simulink model "North_Country_Grid"  (R2025a)
settings: Solver=VariableStepAuto  StartTime=0.0  StopTime=10  RelTol=1e-3
PreLoadFcn:
  | Ts=50e-6;
InitFcn:
  | xInitial = WindFarmType4AverageModelInit;
  | Ts=50e-6;
undefined symbols (not defined in the file): D1, D11, Delta, DiscIntNeverNeededParam, find_system, Fnom_I, Fnom_R, Idc_nom, lagging, level, pulse, test_alpha, Vdc_nom, VLL_nom_I, VLL_nom_R
libraries: spsSecondOrderFilterLib x47, powerlib_extras x38, simulink x34, spsThreePhaseVIMeasurementLib x30, spsFirstOrderFilterLib x29, simulink_extras x26, spsabctodq0Lib x25, spsThreePhaseTransformerTwoWindingsLib x19, spsThreePhaseBreakerLib x18, spsThreePhasePISectionLineLib x17, spsControlledVoltageSourceLib x15, spsOnDelayLib x12
(part 3 of 18)

== system North_Country_Grid/Noble Ellenburg (Type 4, 81 MW) ==
  1 km collector line : spsThreePhasePISectionLineLib/Three-Phase PI Section Line  LConnTagsString=a|b|c  RConnTagsString=A|B|C  Length=1  Frequency=60  Resistances=[ 0.01273 0.3864]  Inductances="[ 0.9337e-3  4.1264e-3]"  Capacitances=[12.74e-9 7.751e-9]
  34.5 kV/ 690V 400 MVA : spsThreePhaseTransformerTwoWindingsLib/Three-Phase Transformer (Two Windings)  Winding1Connection=Delta (D11)  Winding2Connection=Yg  CoreType=Three single-phase transformers  SetSaturation=off  Hysteresis=off  DataFile='hysteresis'  SetInitialFlux=off  Measurements=None  UNITS=pu  NominalPower="[400e6  60]"  Winding1=[34.5e3 , 0.0125 , 0.025]  Winding2=[690, 0.0125, 0.025]  Rm=500  Lm=inf  L0=0.5  Saturation=[ 0,0 ; 0.0024,1.2 ; 1.0,1.52 ]  InitialFluxes=[ 0.8 , -0.8 , 0.7 ]  BreakLoop=off  DiscreteSolver=Trapezoidal iterative  DataType=off  TransfoNumber=0
  345kV/34.5 kV 400 MVA : spsThreePhaseTransformerTwoWindingsLib/Three-Phase Transformer (Two Windings)  Winding1Connection=Delta (D11)  Winding2Connection=Yg  CoreType=Three single-phase transformers  SetSaturation=off  Hysteresis=off  DataFile='basic_model'  SetInitialFlux=off  Measurements=None  UNITS=pu  NominalPower=[400e6 60 ]  Winding1="[ 345e3  0.0125   0.025 ]"  Winding2="[34.5e3  0.0125  0.025]"  Rm=500  Lm=inf  L0=0.5  Saturation="[ 0,0  ;  0.005,1.2  ;  1.0,1.4 ]"  InitialFluxes=[ 0.8 , -0.8 , 0.7 ]  BreakLoop=off  DiscreteSolver=Trapezoidal iterative  DataType=off  TransfoNumber=0
  B6 (690 V) : spsThreePhaseVIMeasurementLib/Three-Phase V-I Measurement  VoltageMeasurement=phase-to-ground  SetLabelV=on  LabelV=Vabc_B6  Vpu=on  VpuLL=off  CurrentMeasurement=yes  SetLabelI=on  LabelI=Iabc_B6  Ipu=on  Pbase=5*2e6/0.9  Vbase=690  OutputType=Complex  PhasorSimulation=off  PSBequivalent=0
  Bus Selector : BusSelector  OutputSignals=Vdc_V,wr_pu,PQ_pu.P_pu,PQ_pu.Q_pu
  Constant : Constant  Value=15
  Constant1 : Constant  Value=0
  Demux : Demux  Outputs=2
  MW : Gain  Gain=54*1.5  SaturateOnIntegerOverflow=on  OutDataTypeStr=Inherit: Same as input  ParamDataTypeStr=Inherit: Same as input
  Mux : Mux  Inputs=2
  Wind Farm : Subsystem  LoadFcn=%find_system(gcs,'FollowLinks', 'on', 'LookUnderMasks', 'all');  mask(Wind Turbine: Model 7){Nb_wt=54, ShowParameters=Control parameters for 1 wind turbine, nom=[1.5e6 690 60], Reactances=[ 1.305, 0.296, 0.252, 0.474,  0.243,  0.18 ], Time_constants=[  4.49  0.0681  0.0513  ], Resistance=0.006, mec=[0.62 0.01 1], init=[ 0  0  0  0  0  0  0  0  1 ], Vnom=690, Imax_grid_conv=1.1, RL_grid=[ 0.15 0.15/50], C_var_filter1=150e3, Vdc_nom=1100, C_DClink1=90000e-6, L_R_Boost=[0.0012     5e-3], Pmec1=2e6, wind_speed_CpMax=11, wind0=11, DisplayTurbChar=off, H_WT=4.32, Ksh=0.3, D_mutual=1.5, w_wt0=1, torque0=1, Kdc=[1.1   27.5], Ki_var_reg=0.05, Ki_volt_reg=2, Kgrid_side_cur_reg=[1  50], Kspeed=[5 1], Kboost_cur_reg=[0.025 100], Kp_pitch=15, Kcompensation=[1.5  6], Kfield=[10  20], pitch_max=27, pitch_rate=10, Ts=Ts}
      mask prompts: Nb_wt "Number of wind turbines:"; ShowParameters "Display:"; nom "Nom. power, L-L volt. and freq.: [Pn (VA), Vn (Vrms), fn (Hz)]"; Reactances "Reactances [Xd Xd' Xd'' Xq Xq'' Xl] (p.u.):"; Time_constants "Time constants [Tdo' Tdo'' Tq''] (s):"; Resistance "Resistance Rs (p.u.):"; mec "Inertia constant, friction factor, and pairs of poles: [ H(s)  F(p.u.)  p ]"; init "Initial conditions: [dw(%) th(deg) ia,ib,ic(pu) pha,phb,phc(deg) Vf(pu)]:"; Vnom "Grid-side converter nominal AC voltage (V):"; Imax_grid_conv "Grid-side converter maximum AC current (pu based on generator power and converter nominal AC voltage):"; RL_grid "Grid-side coupling inductor [ L(pu) R(pu),pu based on generator power and converter nominal AC voltage] :"; C_var_filter1 "Line filter capacitor (Q=50) (var):"; Vdc_nom "Nominal DC bus voltage (V)"; C_DClink1 "DC bus capacitor (F):"; L_R_Boost "Boost converter inductance [L(H) R(ohm)]:"; Pmec1 "Nominal mechanical output power (W):"; wind_speed_CpMax "Wind speed at nominal speed and at Cp max (must be between 6 m/s and 30 m/s) (m/s):"; wind0 "Initial wind speed (m/s):"; DisplayTurbChar "Display wind turbine power characteristics:"; H_WT "Wind turbine inertia constant H (s):"; Ksh "Shaft spring constant refer to high-speed shaft (pu of nominal mechanical torque/rad):"; D_mutual "Shaft mutual damping (pu of nominal mechanical torque/pu dw):"; w_wt0 "Turbine initial speed (pu of nominal speed):"; torque0 "Initial output torque (pu of nominal mechanical torque):"; Kdc "DC bus voltage regulator gains [Kp Ki]:"; Ki_var_reg "Grid-side converter var regulator gain [ Ki]:"; Ki_volt_reg "Grid-side converter voltage regulator gain [ Ki]:"; Kgrid_side_cur_reg "Grid-side converter current regulator gains [Kp Ki]:"; Kspeed "Speed regulator gains [Kp Ki]:"; Kboost_cur_reg "Boost inductor current regulator gains [Kp Ki]:"; Kp_pitch "Pitch controller gain [Kp]:"; Kcompensation "Pitch compensation gains [Kp Ki]:"; Kfield "Field excitation gains [Kp Ki]:"; pitch_max "Maximum pitch angle (deg):"; pitch_rate "Maximum rate of change of pitch angle (deg/s)"; Ts "Sample time (s):"
      mask help: This block implements a model of a variable speed pitch controlled wind turbine using a synchronous generator.
      mask init: same as North_Country_Grid/Marble River (Type 4, 215.25 MW)/Wind Farm
      mask TypeOptions ShowParameters: Generator data for 1 wind turbine | Converters data for 1 wind turbine | Turbine data for 1 wind turbine | Drive train data for 1 wind turbine | Control parameters for 1 wind turbine
      mask Callback ShowParameters:
      | BlockName=getfullname(gcb);
      | %
      | Param_Show=get_param(BlockName,'ShowParameters');
      | Param_DisplayTurbChar=get_param(BlockName,'DisplayTurbChar');
      | 
      | p_mask{3}='off';p_mask{4}='off';p_mask{5}='off';
      | p_mask{6}='off';p_mask{7}='off';p_mask{8}='off';p_mask{9}='off';
      | p_mask{10}='off';p_mask{11}='off';p_mask{12}='off';p_mask{13}='off';
      | p_mask{14}='off';p_mask{15}='off';p_mask{16}='off';p_mask{17}='off';
      | p_mask{18}='off';p_mask{19}='off';p_mask{20}='off';p_mask{21}='off';
      | p_mask{22}='off';p_mask{23}='off';p_mask{24}='off';p_mask{25}='off';
      | p_mask{26}='off';p_mask{27}='off';p_mask{28}='off';p_mask{29}='off';
      | p_mask{30}='off';p_mask{31}='off';p_mask{32}='off';p_mask{33}='off';
      | p_mask{34}='off';p_mask{35}='off';
      | 
      | switch Param_Show
      | 	case 'Generator data for 1 wind turbine'
      | 		p_mask{3}='on';p_mask{4}='on';p_mask{5}='on';
      |         p_mask{6}='on';p_mask{7}='on';p_mask{8}='on';
      |     case 'Converters data for 1 wind turbine'
      | 		p_mask{9}='on';p_mask{10}='on';p_mask{11}='on';
      |         p_mask{12}='on';p_mask{13}='on';p_mask{14}='on';p_mask{15}='on';
      | 	case 'Turbine data for 1 wind turbine'
      | 		p_mask{16}='on';p_mask{17}='on';p_mask{18}='on';p_mask{19}='on';
      |     case 'Drive train data for 1 wind turbine'
      |         p_mask{20}='on';p_mask{21}='on';p_mask{22}='on';p_mask{23}='on';
      |         p_mask{24}='on';
      |     case 'Control parameters for 1 wind turbine'
      |         p_mask{25}='on';p_mask{26}='on';p_mask{27}='on';
      |         p_mask{28}='on';p_mask{29}='on';p_mask{30}='on';p_mask{31}='on';
      |         p_mask{32}='on';p_mask{33}='on';p_mask{34}='on';p_mask{35}='on';
      | end
      | 
      | ParVisible={'on','on',p_mask{3},p_mask{4},p_mask{5},p_mask{6},...
      |     p_mask{7},p_mask{8},p_mask{9},p_mask{10},p_mask{11},p_mask{12},...
      |     p_mask{13},p_mask{14},p_mask{15},p_mask{16},p_mask{17},p_mask{18},...
      |     p_mask{19},p_mask{20},p_mask{21},p_mask{22},p_mask{23},p_mask{24},...
      |     p_mask{25},p_mask{26},p_mask{27},p_mask{28},p_mask{29},p_mask{30},...
      |     p_mask{31},p_mask{32},p_mask{33},p_mask{34},p_mask{35},'on'};
      | %
      | set_param(BlockName,'MaskVisibilities',ParVisible);
      | set_param(BlockName,'DisplayTurbChar',Param_DisplayTurbChar);
      mask Display: disp(' ');
  Wind Farm Scope : Scope  NumInputPorts=6
      settings: ActiveDisplayYMinimum=-6.12469  ActiveDisplayYMaximum=6.81618  DataLoggingSaveFormat=Array
  A : PMIOPort  Side=Left
  B : PMIOPort  Port=2  Side=Left
  C : PMIOPort  Port=3  Side=Left
  wires:
  Constant1/1 -> Wind Farm/2(Qref_pu)
  [Vabc_B6] -> Wind Farm Scope/1  "Vabc_B575 (pu)"
  Demux/1 -> Wind Farm Scope/5  "P (MW)"
  Bus Selector/1 -> Wind Farm Scope/3  "<Vdc_V>"
  Demux/2 -> Wind Farm Scope/6  "Q (Mvar)"
  Mux/1 -> MW/1
  Bus Selector/2 -> Wind Farm Scope/4  "<wr_pu>"
  Wind Farm/1(m) -> Bus Selector/1
  Bus Selector/3 -> Mux/1  "<P_pu>"
  Bus Selector/4 -> Mux/2  "<Q_pu>"
  MW/1 -> Demux/1
  [Iabc_B6] -> Wind Farm Scope/2  "Iabc_B575 (pu)"
  Constant/1 -> Wind Farm/1("Wind (m/s) ")
  connections:
  34.5 kV/ 690V 400 MVA/RConn2 -- B6 (690 V)/LConn2
  B6 (690 V)/RConn1 -- Wind Farm/LConn1
  34.5 kV/ 690V 400 MVA/RConn1 -- B6 (690 V)/LConn1
  34.5 kV/ 690V 400 MVA/RConn3 -- B6 (690 V)/LConn3
  B6 (690 V)/RConn3 -- Wind Farm/LConn3
  Wind Farm/LConn2 -- B6 (690 V)/RConn2
  345kV/34.5 kV 400 MVA/LConn3 -- C/RConn1
  345kV/34.5 kV 400 MVA/LConn1 -- A/RConn1
  345kV/34.5 kV 400 MVA/LConn2 -- B/RConn1
  1 km collector line/LConn2 -- 345kV/34.5 kV 400 MVA/RConn2
  1 km collector line/LConn1 -- 345kV/34.5 kV 400 MVA/RConn1
  1 km collector line/RConn1 -- 34.5 kV/ 690V 400 MVA/LConn1
  1 km collector line/RConn2 -- 34.5 kV/ 690V 400 MVA/LConn2
  1 km collector line/RConn3 -- 34.5 kV/ 690V 400 MVA/LConn3
  1 km collector line/LConn3 -- 345kV/34.5 kV 400 MVA/RConn3

== system North_Country_Grid/St. Lawrence-FDR Power Dam 1 ==
  345 kV/20 kV 1000 MVA : spsThreePhaseTransformerTwoWindingsLib/Three-Phase Transformer (Two Windings)  Winding1Connection=Delta (D11)  Winding2Connection=Yg  CoreType=Three single-phase transformers  SetSaturation=off  Hysteresis=off  DataFile='basic_model'  SetInitialFlux=off  Measurements=None  UNITS=pu  NominalPower=[1000e6 60 ]  Winding1="[ 345e3  0.0125   0.025 ]"  Winding2="[ 20e3  0.0125  0.025]"  Rm=500  Lm=500  L0=0.5  Saturation="[ 0,0  ;  0.005,1.2  ;  1.0,1.4 ]"  InitialFluxes=[ 0.8 , -0.8 , 0.7 ]  BreakLoop=off  DiscreteSolver=Trapezoidal iterative  DataType=off  TransfoNumber=0
  Bus Selector : BusSelector  OutputSignals="dq0 components.Stator voltage  vq (pu),dq0 components.Stator voltage  vd (pu),Mechanical.Rotor speed  wm  (pu),Mechanical.Rotor speed deviation  dw (pu),Output active power   Peo (pu)"
  Constant : Constant
  Constant1 : Constant
  Constant2 : Constant
  Excitation System : spsExcitationSystemLib/Excitation System  tr=20e-3  reg=[300, 0.001]  exc=[ 1, 0 ]  tgr=[ 0, 0 ]  damp=[ 0.001, 0.1 ]  sat=[ 0, 0 ]  lim=[ -11.5, 11.5, 0 ]  v0=[1 2.1284]
  Ground : Ground
  Hydraulic Turbine and Governor : spsHydraulicTurbineandGovernorLib/Hydraulic Turbine and Governor  sm="[ 10/3  0.07 ]"  gate="[  0.01  0.97518  -0.1  0.1 ]"  reg="[  0.05  1.163 0.105  0  0.01  ]"  hyd="[  0 1 ]"  dref=0  po=1.0094
  Power Dam Turbines 1-8 : spsSynchronousMachinepuStandardLib/Synchronous Machine pu Standard  PresetModel=No  MechanicalLoad=Mechanical power Pm  ShowDetailedParameters=on  RotorType=Salient-pole  Units=per unit standard parameters  MeasurementBus=off  NominalParameters=[456e+06 20e+03 60]  Reactances1=[ 1.81, 0.3, 0.23, 1.76, 0.65, 0.25, 0.15 ]  Reactances2=[2.24 0.17 0.12 1.02 0.13 0.08]  dAxisTimeConstants=Short-circuit  qAxisTimeConstants=Short-circuit  TimeConstants1="[ 4.4849  0.0681  0.1  ]"  TimeConstants2=[ 8.0, 0.03, 1.0, 0.07 ]  TimeConstants3="[  4.49  0.0681  0.0513  ]"  TimeConstants4=[ 8.0, 0.03, 0.3371, 0.0295 ]  TimeConstants5=[ 1.01, 0.053, 0.1 ]  TimeConstants6=[ 1.3201, 0.023, 1.0, 0.07 ]  TimeConstants7=[0.12 0.006 0.006]  TimeConstants8=[ 1.3201, 0.0231, 0.3371, 0.0295 ]  StatorResistance=0.037875  Mechanical=[1.028 0.02056 2]  PolePairs=20  InitialConditions=[0 -55.1392 1.01711 1.01711 1.01711 -5.05639 -125.056 114.944 2.12836]  SetSaturation=on  Saturation=[0.6404,0.7127,0.8441,0.9214,0.9956,1.082,1.19,1.316,1.457;0.7,0.7698,0.8872,0.9466,0.9969,1.046,1.1,1.151,1.201]  LoadFlowParameters=[1 912000000 0 0 0]  TsPowergui=0  TsBlock=-1  IterativeModel=Trapezoidal non iterative  IterativeDiscreteModel=Trapezoidal non iterative  BusType=PV  Pref=456000000  Qref=0  Qmin=-Inf  Qmax=Inf  PLF=0  QLF=0
  Terminator : Terminator
  Three-Phase Parallel RLC Load : spsThreePhaseParallelRLCLoadLib/Three-Phase Parallel RLC Load  LConnTagsString=A|B|C  Configuration=Y (grounded)  NominalVoltage=20e3  Vabc=[1e3 1e3 1e3]  Vabcp=[1e3 1e3 1e3]  NominalFrequency=60  UnbalancedPower=off  ActivePower=1e3  InductivePower=0  CapacitivePower=0  Pabc=[10e3 9e3 11e3]  QLabc=[100 90 110]  QCabc=[100 90 110]  Pabcp=[10e3 9e3 11e3]  QLabcp=[100 90 110]  QCabcp=[100 90 110]  Measurements=None  LoadType=constant Z
  A : PMIOPort  Side=Left
  B : PMIOPort  Port=2  Side=Left
  C : PMIOPort  Port=3  Side=Left
  tag scope: Dam1Rotor=global
  wires:
  Excitation System/1 -> Power Dam Turbines 1-8/2
  Constant/1 -> Excitation System/1
  Bus Selector/5 -> Hydraulic Turbine and Governor/4  "<Output active power   Peo (pu)>"
  Bus Selector/3 -> [Dam1Rotor], Hydraulic Turbine and Governor/3  "<Rotor speed  wm  (pu)>"
  Bus Selector/2 -> Excitation System/2  "<Stator voltage  vd (pu)>"
  Power Dam Turbines 1-8/1 -> Bus Selector/1
  Bus Selector/1 -> Excitation System/3  "<Stator voltage  vq (pu)>"
  Hydraulic Turbine and Governor/1 -> Power Dam Turbines 1-8/1
  Constant2/1 -> Hydraulic Turbine and Governor/2
  Bus Selector/4 -> Hydraulic Turbine and Governor/5  "<Rotor speed deviation  dw (pu)>"
  Constant1/1 -> Hydraulic Turbine and Governor/1
  Hydraulic Turbine and Governor/2 -> Terminator/1
  Ground/1 -> Excitation System/4
  connections:
  345 kV/20 kV 1000 MVA/LConn1 -- A/RConn1
  345 kV/20 kV 1000 MVA/RConn2 -- Three-Phase Parallel RLC Load/LConn2 -- Power Dam Turbines 1-8/RConn2
  345 kV/20 kV 1000 MVA/LConn2 -- B/RConn1
  345 kV/20 kV 1000 MVA/RConn1 -- Three-Phase Parallel RLC Load/LConn1 -- Power Dam Turbines 1-8/RConn1
  345 kV/20 kV 1000 MVA/LConn3 -- C/RConn1
  345 kV/20 kV 1000 MVA/RConn3 -- Three-Phase Parallel RLC Load/LConn3 -- Power Dam Turbines 1-8/RConn3

== system North_Country_Grid/St. Lawrence-FDR Power Dam 2 ==
  345 kV/20 kV 1000 MVA : spsThreePhaseTransformerTwoWindingsLib/Three-Phase Transformer (Two Windings)  Winding1Connection=Delta (D11)  Winding2Connection=Yg  CoreType=Three single-phase transformers  SetSaturation=off  Hysteresis=off  DataFile='basic_model'  SetInitialFlux=off  Measurements=None  UNITS=pu  NominalPower=[1000e6 60 ]  Winding1="[ 345e3  0.0125   0.025 ]"  Winding2="[ 20e3  0.0125  0.025]"  Rm=500  Lm=500  L0=0.5  Saturation="[ 0,0  ;  0.005,1.2  ;  1.0,1.4 ]"  InitialFluxes=[ 0.8 , -0.8 , 0.7 ]  BreakLoop=off  DiscreteSolver=Trapezoidal iterative  DataType=off  TransfoNumber=0
  Bus Selector : BusSelector  OutputSignals="dq0 components.Stator voltage  vq (pu),dq0 components.Stator voltage  vd (pu),Mechanical.Rotor speed  wm  (pu),Mechanical.Rotor speed deviation  dw (pu),Output active power   Peo (pu)"
  Constant : Constant
  Constant1 : Constant
  Constant2 : Constant
  Excitation System : spsExcitationSystemLib/Excitation System  tr=20e-3  reg=[300 0.001]  exc=[ 1, 0 ]  tgr=[ 0, 0 ]  damp=[ 0.001, 0.1 ]  sat=[ 0, 0 ]  lim=[ -11.5, 11.5, 0 ]  v0=[1 2.1284]
  Ground : Ground
  Hydraulic Turbine and Governor : spsHydraulicTurbineandGovernorLib/Hydraulic Turbine and Governor  sm="[ 10/3  0.07 ]"  gate="[  0.01  0.97518  -0.1  0.1 ]"  reg="[  0.05  1.163 0.105  0  0.01  ]"  hyd="[  0  2.67 ]"  dref=0  po=1.0094
  Power Dam Turbines 9-16 : spsSynchronousMachinepuStandardLib/Synchronous Machine pu Standard  PresetModel=No  MechanicalLoad=Mechanical power Pm  ShowDetailedParameters=on  RotorType=Salient-pole  Units=per unit standard parameters  MeasurementBus=off  NominalParameters=[456e+06 20e+03 60]  Reactances1=[ 1.81, 0.3, 0.23, 1.76, 0.65, 0.25, 0.15 ]  Reactances2=[2.24 0.17 0.12 1.02 0.13 0.08]  dAxisTimeConstants=Short-circuit  qAxisTimeConstants=Short-circuit  TimeConstants1="[ 4.4849  0.0681  0.1  ]"  TimeConstants2=[ 8.0, 0.03, 1.0, 0.07 ]  TimeConstants3="[  4.49  0.0681  0.0513  ]"  TimeConstants4=[ 8.0, 0.03, 0.3371, 0.0295 ]  TimeConstants5=[ 1.01, 0.053, 0.1 ]  TimeConstants6=[ 1.3201, 0.023, 1.0, 0.07 ]  TimeConstants7=[0.12 0.006 0.006]  TimeConstants8=[ 1.3201, 0.0231, 0.3371, 0.0295 ]  StatorResistance=0.037875  Mechanical=[1.028 0.02056 2]  PolePairs=20  InitialConditions=[0 -55.1393 1.01711 1.01711 1.01711 -5.05641 -125.056 114.944 2.12836]  SetSaturation=on  Saturation=[0.6404,0.7127,0.8441,0.9214,0.9956,1.082,1.19,1.316,1.457;0.7,0.7698,0.8872,0.9466,0.9969,1.046,1.1,1.151,1.201]  LoadFlowParameters=[1 912000000 0 0 0]  TsPowergui=0  TsBlock=-1  IterativeModel=Trapezoidal non iterative  IterativeDiscreteModel=Trapezoidal non iterative  BusType=PV  Pref=456000000  Qref=0  Qmin=-Inf  Qmax=Inf  PLF=0  QLF=0
  Terminator : Terminator
  Three-Phase Parallel RLC Load : spsThreePhaseParallelRLCLoadLib/Three-Phase Parallel RLC Load  LConnTagsString=A|B|C  Configuration=Y (grounded)  NominalVoltage=20e3  Vabc=[1e3 1e3 1e3]  Vabcp=[1e3 1e3 1e3]  NominalFrequency=60  UnbalancedPower=off  ActivePower=1e3  InductivePower=0  CapacitivePower=0  Pabc=[10e3 9e3 11e3]  QLabc=[100 90 110]  QCabc=[100 90 110]  Pabcp=[10e3 9e3 11e3]  QLabcp=[100 90 110]  QCabcp=[100 90 110]  Measurements=None  LoadType=constant Z
  A : PMIOPort  Side=Left
  B : PMIOPort  Port=2  Side=Left
  C : PMIOPort  Port=3  Side=Left
  tag scope: Dam2Rotor=global
  wires:
  Excitation System/1 -> Power Dam Turbines 9-16/2
  Constant/1 -> Excitation System/1
  Bus Selector/5 -> Hydraulic Turbine and Governor/4  "<Output active power   Peo (pu)>"
  Bus Selector/3 -> [Dam2Rotor], Hydraulic Turbine and Governor/3  "<Rotor speed  wm  (pu)>"
  Bus Selector/2 -> Excitation System/2  "<Stator voltage  vd (pu)>"
  Power Dam Turbines 9-16/1 -> Bus Selector/1
  Bus Selector/1 -> Excitation System/3  "<Stator voltage  vq (pu)>"
  Hydraulic Turbine and Governor/1 -> Power Dam Turbines 9-16/1
  Constant2/1 -> Hydraulic Turbine and Governor/2
  Bus Selector/4 -> Hydraulic Turbine and Governor/5  "<Rotor speed deviation  dw (pu)>"
  Constant1/1 -> Hydraulic Turbine and Governor/1
  Hydraulic Turbine and Governor/2 -> Terminator/1
  Ground/1 -> Excitation System/4
  connections:
  345 kV/20 kV 1000 MVA/LConn1 -- A/RConn1
  345 kV/20 kV 1000 MVA/RConn2 -- Three-Phase Parallel RLC Load/LConn2 -- Power Dam Turbines 9-16/RConn2
  345 kV/20 kV 1000 MVA/LConn2 -- B/RConn1
  345 kV/20 kV 1000 MVA/RConn1 -- Three-Phase Parallel RLC Load/LConn1 -- Power Dam Turbines 9-16/RConn1
  345 kV/20 kV 1000 MVA/LConn3 -- C/RConn1
  345 kV/20 kV 1000 MVA/RConn3 -- Three-Phase Parallel RLC Load/LConn3 -- Power Dam Turbines 9-16/RConn3

== system North_Country_Grid/Willis Substation ==
  Constant{,1..4} (5 alike) : Constant
  Three-Phase Breaker{,1..4} (5 alike) : spsThreePhaseBreakerLib/Three-Phase Breaker  InitialState=closed  SwitchA=on  SwitchB=on  SwitchC=on  SwitchTimes="[1/60  5/60]"  External=on  BreakerResistance=0.01  SnubberResistance=1e6  SnubberCapacitance=inf  Measurements=None
  a : PMIOPort  Side=Right
  A : PMIOPort  Port=2  Side=Left
  B : PMIOPort  Port=3  Side=Left
  b : PMIOPort  Port=4  Side=Right
  C : PMIOPort  Port=5  Side=Left
  c : PMIOPort  Port=6  Side=Right
  a1 : PMIOPort  Port=7  Side=Right
  A1 : PMIOPort  Port=8  Side=Left
  b1 : PMIOPort  Port=9  Side=Right
  B1 : PMIOPort  Port=10  Side=Left
  C1 : PMIOPort  Port=11  Side=Left
  c1 : PMIOPort  Port=12  Side=Right
  wires:
  Constant/1 -> Three-Phase Breaker/1
  Constant2/1 -> Three-Phase Breaker2/1
  Constant1/1 -> Three-Phase Breaker1/1
  Constant4/1 -> Three-Phase Breaker4/1
  Constant3/1 -> Three-Phase Breaker3/1
  connections:
  Three-Phase Breaker1/LConn3 -- C/RConn1
  Three-Phase Breaker1/LConn1 -- A/RConn1
  Three-Phase Breaker2/LConn1 -- A1/RConn1
  Three-Phase Breaker/RConn3 -- c/RConn1
  Three-Phase Breaker3/RConn3 -- c1/RConn1
  Three-Phase Breaker/RConn2 -- b/RConn1
  Three-Phase Breaker1/LConn2 -- B/RConn1
  Three-Phase Breaker1/RConn2 -- Three-Phase Breaker4/LConn2 -- Three-Phase Breaker/LConn2
  Three-Phase Breaker2/RConn3 -- Three-Phase Breaker3/LConn3 -- Three-Phase Breaker4/RConn3
  Three-Phase Breaker2/LConn3 -- C1/RConn1
  Three-Phase Breaker/RConn1 -- a/RConn1
  Three-Phase Breaker2/RConn1 -- Three-Phase Breaker4/RConn1 -- Three-Phase Breaker3/LConn1
  Three-Phase Breaker3/RConn2 -- b1/RConn1
  Three-Phase Breaker3/LConn2 -- Three-Phase Breaker4/RConn2 -- Three-Phase Breaker2/RConn2
  Three-Phase Breaker1/RConn3 -- Three-Phase Breaker/LConn3 -- Three-Phase Breaker4/LConn3
  Three-Phase Breaker2/LConn2 -- B1/RConn1
  Three-Phase Breaker3/RConn1 -- a1/RConn1
  Three-Phase Breaker1/RConn1 -- Three-Phase Breaker/LConn1 -- Three-Phase Breaker4/LConn1

== system North_Country_Grid/Chateauguay HVDC Back-to-Back Converter/Data Acquisition ==
  AC_INVERTER : Scope  NumInputPorts=2
      settings: DataLoggingSaveFormat=Array
  AC_RECTIFIER : Scope  NumInputPorts=2
      settings: DataLoggingSaveFormat=Array
  Demux : Demux  Outputs=2
      settings: DisplayOption=none
  Demux1 : Demux  Outputs=[1 2]
      settings: DisplayOption=none
  FAULT : Scope  NumInputPorts=2
      settings: DataLoggingSaveFormat=Array
  INVERTER : Scope  NumInputPorts=5
      settings: DataLoggingSaveFormat=Array
  Multimeter : spsMultimeterLib/Multimeter  Tag=PoWeRsYsTeMmEaSuReMeNt  L=44  sel=[24 23]  yselected={}  Gain=[1 1]  OutputType=Magnitude  PlotAtSimulationStop=off  PhasorSimulation=off
      settings: AttributesFormatString=\n
  Multimeter1 : spsMultimeterLib/Multimeter  Tag=PoWeRsYsTeMmEaSuReMeNt  L=44  sel=[11 37 39]  yselected={}  Gain=[1 1 1]  OutputType=Magnitude  PlotAtSimulationStop=off  PhasorSimulation=off
      settings: AttributesFormatString=\n
  Multimeter2 : spsMultimeterLib/Multimeter  Tag=PoWeRsYsTeMmEaSuReMeNt  L=44  sel=1  yselected={}  Gain=1  OutputType=Magnitude  PlotAtSimulationStop=off  PhasorSimulation=off
      settings: AttributesFormatString=\n
  Mux{,1..4} (5 alike) : Mux  Inputs=2
  PROTECTION INVERTER : Scope  NumInputPorts=2
      settings: DataLoggingSaveFormat=Array
  PROTECTION RECTIFIER : Scope  NumInputPorts=2
      settings: DataLoggingSaveFormat=Array
  RECTIFIER : Scope  NumInputPorts=4
      settings: DataLoggingSaveFormat=Array
  Terminator : Terminator
  VALVE13_RECT : Scope  NumInputPorts=3
      settings: DataLoggingSaveFormat=Array
  VALVE1_INV : Scope  NumInputPorts=3
      settings: DataLoggingSaveFormat=Array
  wires:
  [Mode_R] -> RECTIFIER/4  "Control Mode:   0=blocked  1=current 2=voltage 3=alpha min  4=alpha max 5=forced alpha 6=gamma"
  Demux/2 -> FAULT/2  "I DC Fault (A)"
  Demux/1 -> FAULT/1  "I AC Fault (A)"
  [alpha_ord_I] -> INVERTER/3  "alpha_ord (deg)"
  [Iabc_I] -> AC_INVERTER/2  "Iabc (pu/100MVA)"
  [Vabc_I] -> AC_INVERTER/1  "Vabc (pu)"
  [alpha_ord_R] -> RECTIFIER/3  "alpha_ord (deg)"
  [VdL_R] -> RECTIFIER/1  "VdL (pu)"
  [Iabc_R] -> AC_RECTIFIER/2  "Iabc (pu/100 MVA)"
  [Vabc_R] -> AC_RECTIFIER/1  "Vabc  (pu)"
  Multimeter/1 -> Demux/1
  [Low_ac_volt_I] -> PROTECTION INVERTER/1  "Low_ac_volt_I"
  [A_min_I] -> PROTECTION INVERTER/2  "A_min_I"
  [Low_ac_volt_R] -> PROTECTION RECTIFIER/1  "Low_ac_volt_R"
  Mux/1 -> RECTIFIER/2  "Id  Idref _lim(pu)"
  [Id_R] -> Mux/1
  [Id_ref_lim_R] -> Mux/2
  [Id_I] -> Mux1/1
  [Id_ref_lim_I] -> Mux1/2
  Mux1/1 -> INVERTER/2  "Id Idref _lim(pu)"
  [Mode_I] -> INVERTER/4  "Control Mode:  0=blocked  1=current  2=voltage  3=alpha min  4=alpha max  5=forced alpha  6=gamma"
  [VdL_I] -> Mux2/1  "VdL (pu)"
  Mux2/1 -> INVERTER/1  "VdL  Vd_ref (pu)"
  [Vd_ref_I] -> Mux2/2
  [Gamma_mean] -> Mux3/1
  Mux3/1 -> INVERTER/5  "gamma_mean  gamma_ref (deg)"
  [Forced_alpha_R] -> PROTECTION RECTIFIER/2  "Forced_alpha_R"
  Multimeter1/1 -> Demux1/1
  Demux1/1 -> VALVE13_RECT/1  "uSw1 (V)"
  Demux1/2 -> VALVE13_RECT/2  "iSw1 & Sw3 (A)"
  [alpha_ord_R] -> VALVE13_RECT/3  "alpha_ord (deg)"
  Multimeter2/1 -> VALVE1_INV/1  "uSw1 (V)"
  Mux4/1 -> VALVE1_INV/2  "iSw1  Ucom1 (pu)"
  [ISw1Y_pu] -> Mux4/1
  [Ucom1Y_pu] -> Mux4/2
  [Gamma_ref_I] -> Mux3/2
  [Gamma_mean] -> VALVE1_INV/3  "gamma mean (deg)"
  [gamma_min_I] -> Terminator/1

== system North_Country_Grid/Chateauguay HVDC Back-to-Back Converter/Inverter ==
  1200 MVA : spsThreePhaseTransformerThreeWindingsLib/Three-Phase Transformer (Three Windings)  Winding1Connection=Yg  Winding2Connection=Y  Winding3Connection=Delta (D1)  CoreType=Three single-phase transformers  SetSaturation=off  Hysteresis=off  DataFile='hysteresis'  SetInitialFlux=off  Measurements=None  UNITS=pu  NominalPower=[ 1200e6 , 50 ]  Winding1="[VLL_nom_I*0.96 0.0025  0 ]"  Winding2="[ 200e3  0.0025 0.24]"  Winding3=[ 200e3 0.0025 0.24 ]  Rm=500  Lm=500  L0=0.5  Saturation="[0 0; 0.0024 1.2; 1.0  1.45]"  InitialFluxes=[-1.10749033878531 0.564800371868647 0.542689966916658]  BreakLoop=off  DiscreteSolver=Trapezoidal iterative  DataType=off  TransfoNumber=0
      settings: AttributesFormatString=\n
  A->pu : Gain  Gain=1/Idc_nom  SaturateOnIntegerOverflow=on  OutDataTypeStr=Inherit: Same as input  ParamDataTypeStr=Inherit: Same as input
  Id : spsCurrentMeasurementLib/Current Measurement  Tag=PoWeRsYsTeMmEaSuReMeNt  PhasorSimulation=off  OutputType=Magnitude  PSBequivalent=0
      settings: AttributesFormatString=\n
  Inverter : Subsystem
      mask Display: plot(0,0,100,100,[30 70 50 30 ], [60 60 40 60], [50 50], [25 40], [50 50], [ 60 75], [30 70], [40 40], [50 60 70], [40 30 30]);
  Zinv : spsImpedanceMeasurementLib/Impedance Measurement  LConnTagsString=+|-  Factor=1/2
  A : PMIOPort  Side=Left
  B : PMIOPort  Port=2  Side=Left
  C : PMIOPort  Port=3  Side=Left
  + : PMIOPort  Port=4  Side=Right
  - : PMIOPort  Port=5  Side=Right
  tag scope: Id_I=global
  wires:
  [PulsesY_I] -> Inverter/1(Py)
  [PulsesD_I] -> Inverter/2(Pd)
  Id/1 -> A->pu/1
  A->pu/1 -> [Id_I]
  connections:
  C/RConn1 -- 1200 MVA/LConn3
  A/RConn1 -- Zinv/LConn1 -- 1200 MVA/LConn1
  -/RConn1 -- Inverter/RConn2
  Inverter/LConn6 -- 1200 MVA/RConn6
  1200 MVA/RConn5 -- Inverter/LConn5
  Inverter/LConn4 -- 1200 MVA/RConn4
  1200 MVA/RConn3 -- Inverter/LConn3
  Inverter/LConn2 -- 1200 MVA/RConn2
  1200 MVA/RConn1 -- Inverter/LConn1
  1200 MVA/LConn2 -- Zinv/LConn2 -- B/RConn1
  +/RConn1 -- Id/LConn1
  Id/RConn1 -- Inverter/RConn1

== system North_Country_Grid/Chateauguay HVDC Back-to-Back Converter/Inverter Control and Protection ==
  note: Block/Deblock sequence
  12-pulse Firing Control : Subsystem  mask(HVDC Discrete 12-pulse Firing Control){Pw=101.5, PLL_PF=[0,  Fnom_I], PLL_G=[60, 1400], dt=Ts}
      mask prompts: Pw "{Pulse Generator}: Pulse Width (deg)"; PLL_PF "{PLL}: Initial [Phase (deg) Frequency (Hz)]"; PLL_G "{PLL}: Regulator gains [Kp (rad)  Ki (rad/s)]"; dt "Sample Time (s):"
      mask help:
      | This block contains a PLL and a 12-pulse generator to provide the firing pulses to the HVDC converter.
      | The firing control is of the equidistant type. It is based on a Phase Locked Loop (PLL) synchronized on positive-sequence of the fundamental voltage.
      mask init:
      | PLL_ph = PLL_PF(1); PLL_f0 = PLL_PF(2);
      | PLL_Kp = PLL_G(1); PLL_Ki = PLL_G(2);
      mask Help:
      | INPUTS:
      | alpha :  Desired firing angle of thyristors (deg).
      | Vabc  : 3 phase-to-ground voltages (pu)  on the primary winding of the YgYD converter transformer
      | Block  : Logical signal  (0-1). The pulses are not generated when the value is 1.
      | 
      | 
      | 
      | OUTPUTS:
      |  PulsesY :  6 pulses to be sent to the half converter connected to the Wye winding.
      |  PulsesD :  6 pulses to be sent to the half converter connected to the Delta winding.
  Data Type Conversion : DataTypeConversion  OutDataTypeStr=boolean
  Enable Ref.  Voltage Step : ManualSwitch
  Enable Ref. Gamma Step : ManualSwitch  CurrentSetting=0
  Gamma Measurement : Subsystem
  Gamma Step : spsStairGeneratorLib/Stair Generator  t="[ 0  0.7  0.9 ]"  e="[ 18   23   18  ]"  Ts=Ts
  Gamma min : Constant  Value=18
  Inverter Pole Control (Current/Voltage/Gamma) : Subsystem  DialogController=POWERSYS.PowerSysDialog  mask(Discrete HVDC Controller){Mode=Inverter (Current + Voltage + Gamma), XPILim=[166, 92], XLin=[160, 120], XKPI_I=[45, 4500, 90], Id_marg=0.1, XKPI_V=[35, 2250,  90], Vd_marg=0.05, XKPI_G=[2, 40,  90 ], G_marg=1, T_I=0.3e-3, XT_V=[15,  0.707], Xvdcol=[0.6, 0.18, 0.30, 0.1, 0.080], alpha_const=off, Xalpha_fix=[92, inf, -1000], Ts=Ts}
      mask prompts: Mode "Control Mode :"; XPILim "{Alpha Limits}  [alpha max (deg), alpha min (deg) ]"; XLin "Kp Lin. Angle Limits (alpha or beta) : [Max  (deg), Min  (deg) ]"; XKPI_I "{Current Regulator}   [Kp (deg/pu) , Ki (deg/pu/s), AlphaInit (deg) ]"; Id_marg "Current Margin (pu) :"; XKPI_V "{Voltage Regulator}   [Kp (deg/pu) , Ki (deg/pu/s),  AlphaInit (deg) ]"; Vd_marg "Voltage Margin (pu):"; XKPI_G "{Gamma Regulator} [Kp, Ki (s), AlphaInit (deg)]"; G_marg "Gamma Margin (deg):"; T_I "{Id Meas. Filter H(s)=1/(1+Ts)} T(s):"; XT_V "{Vd Meas. Low-Pass 2nd Order Filter}  [fo,  Zeta ]"; Xvdcol "{VDCOL}  [ VdThresh.(pu),VdMin(pu),IdMin(pu),IdMinAbs(pu),Tup(s) ]"; alpha_const "Constant alpha mode"; Xalpha_fix "{Ct.  or Forced alpha)}  [Alpha (deg), + Rate limit, - Rate limit (deg/s)]"; Ts "Sample Time (s):"
      mask help:
      | This block contains the regulators and functions to control the firing angle alpha of a HVDC rectifier or inverter.
      |  See the 'HVDC Transmission System' case study of the User's Manual for description of the block functionality.
      mask init:
      | % Max_lin = max(180-Xlin)  Min_lin = min(180-Xlin)
      | 
      | alpha_max = XPILim(1); alpha_min = XPILim(2);
      | alpha_fix = Xalpha_fix(1); PRate_fix = Xalpha_fix(2);NRate_fix = Xalpha_fix(3);
      | Kp_I = XKPI_I(1); Ki_I = XKPI_I(2); ICi_I = XKPI_I(3);
      | Kp_V = XKPI_V(1); Ki_V = XKPI_V(2); ICi_V = XKPI_V(3);
      | Kp_G = XKPI_G(1); Ki_G = XKPI_G(2); ICi_G = XKPI_G(3);
      | f0_V = XT_V(1); Z_V = XT_V(2);
      | 
      | Inverter = Mode > 1;
      | 
      | if (Mode == 1) 
      | 	Id_marg = 0.0;
      | 	Max_lin = 60; Min_lin = 20;
      | else
      | 	Max_lin = 160; Min_lin = 120;
      | end;
      | 
      | 
      | Vd_seuil = Xvdcol(1); Vd_min=Xvdcol(2);Id_min=Xvdcol(3);Id_min_abs=Xvdcol(4);Tup=Xvdcol(5);
      | if strcmp(alpha_const,'on'), test_alpha = true; else, test_alpha = false; end
      | power_initmask();
      mask Help: This block is part of a subset of blocks in the Extras library that does not have documentation associated with it, other than the block mask description.
      mask TypeOptions Mode: Rectifier (Current) | Inverter (Current + Voltage + Gamma) | Inverter (Current + Voltage) | Inverter (Current + Gamma)
      mask Callback Mode:
      | mode=get_param(gcb,'Mode');
      | 
      | cb=get_param(gcb,'MaskVisibilities');
      | 
      | if strcmp(mode,'Rectifier (Current)')
      | 	cb{10}='on';
      |     cb{11} = 'off';
      | 
      | 	 cb{3}='off';
      | 	 cb{5}='off';cb{6}='off';cb{7}='off';cb{8}='off';cb{9}='off';
      |     set_param(gcb,'MaskVisibilities',cb);
      | elseif (strcmp(mode,'Inverter (Current + Voltage + Gamma)'))
      | 	 cb{3}='off';
      | 	 cb{5}='on';cb{6}='on';cb{7}='on';cb{8}='on';cb{9}='on';cb{11} = 'on';
      | 	 set_param(gcb,'MaskVisibilities',cb);
      | elseif (strcmp(mode,'Inverter (Current + Voltage)'))
      | 	 cb{3}='off';
      | 	 cb{5}='on';cb{6}='on';cb{7}='on';cb{8}='off';cb{9}='off'; cb{11} = 'on';
      |      set_param(gcb,'MaskVisibilities',cb);
      | else
      | 	 cb{3}='off';
      | 	 cb{5}='on';cb{6}='off';cb{7}='off';cb{8}='on';cb{9}='on'; cb{11} = 'on';
      | 	 set_param(gcb,'MaskVisibilities',cb);
      | end
      mask Display: disp('')
  Inverter Protections : Subsystem  TreatAsAtomicUnit=on  mask(Protection LACVD a Radisson (cyc = 1 ms)){}
  Monostable (IC=1) : spsMonostableLib/Monostable  EdgeDetect=Rising  PulseDuration=0.15  ic=1  Ts=Ts
  Multimeter1 : spsMultimeterLib/Multimeter  Tag=PoWeRsYsTeMmEaSuReMeNt  L=44  sel=22  yselected={}  Gain=1  OutputType=Magnitude  PlotAtSimulationStop=off  PhasorSimulation=off
      settings: AttributesFormatString=\n
  On Delay (IC=1) : spsOnDelayLib/On Delay  DelayType=On delay  delay=0.1  ic=1  Ts=Ts
  "Thyristor currents D bridge " : spsMultimeterLib/Multimeter  Tag=PoWeRsYsTeMmEaSuReMeNt  L=44  sel=[25 26 27 28 29 30]  yselected={}  Gain=[1 1 1 1 1 1]  OutputType=Magnitude  PlotAtSimulationStop=off  PhasorSimulation=off
      settings: AttributesFormatString=\n
  Thyristor currents Y bridge : spsMultimeterLib/Multimeter  Tag=PoWeRsYsTeMmEaSuReMeNt  L=44  sel=[31 32 33 34 35 36]  yselected={}  Gain=[1 1 1 1 1 1]  OutputType=Magnitude  PlotAtSimulationStop=off  PhasorSimulation=off
      settings: AttributesFormatString=\n
  Unit Delay : UnitDelay  SampleTime=Ts  HasFrameUpgradeWarning=on
  Unit Delay1 : UnitDelay  SampleTime=Ts  HasFrameUpgradeWarning=on
  V->pu : Gain  Gain=1/Vdc_nom  SaturateOnIntegerOverflow=on  OutDataTypeStr=Inherit: Same as input  ParamDataTypeStr=Inherit: Same as input
  Vd_ref : Constant  Value=1.0
  Vd_ref Step : spsStairGeneratorLib/Stair Generator  t="[ 0  1  1.2  ]"  e="[ 1   1.1   1  ]"  Ts=Ts
  tag scope: A_min_I=global, Gamma_mean=global, Gamma_ref_I=global, Id_ref_lim_I=global, Low_ac_volt_I=global, Mode_I=global, PulsesD_I=global, PulsesY_I=global, VdL_I=global, Vd_ref_I=global, alpha_ord_I=global, gamma_min_I=global
  wires:
  Data Type Conversion/1 -> On Delay (IC=1)/1, Monostable (IC=1)/1
  [Stop_I] -> Data Type Conversion/1
  [Vabc_I] -> Inverter Protections/1(Uabc (pu))
  Inverter Protections/2(AMIN_CFPREV) -> Inverter Pole Control (Current/Voltage/Gamma)/9(D_alpha (deg)), [A_min_I]
  Inverter Protections/1(Low_AC_Voltage) -> [Low_ac_volt_I]
  V->pu/1 -> [VdL_I]
  Multimeter1/1 -> V->pu/1  "Vd Line"
  Enable Ref. Gamma Step/1 -> Inverter Pole Control (Current/Voltage/Gamma)/8(gamma_ref (deg)), [Gamma_ref_I]
  Gamma Step/1 -> Enable Ref. Gamma Step/1
  Gamma min/1 -> Enable Ref. Gamma Step/2
  Gamma Measurement/1(gamma_min) -> [gamma_min_I]
  [Vabc_I] -> Gamma Measurement/1(Vabc)
  Gamma Measurement/2(gamma_mean) -> Inverter Pole Control (Current/Voltage/Gamma)/7(gamma_meas (deg)), [Gamma_mean]
  Inverter Pole Control (Current/Voltage/Gamma)/1(alpha_ord (deg)) -> 12-pulse Firing Control/1(alpha_ord (deg)), [alpha_ord_I]
  Inverter Pole Control (Current/Voltage/Gamma)/2(Id_ref_lim) -> [Id_ref_lim_I]
  Inverter Pole Control (Current/Voltage/Gamma)/3(mode) -> [Mode_I]
  [Vabc_I] -> 12-pulse Firing Control/2(Vabc (pu))
  [VdL_I] -> Inverter Pole Control (Current/Voltage/Gamma)/1(VdL (pu))
  [Id_I] -> Inverter Pole Control (Current/Voltage/Gamma)/2(Id (pu))
  [Id_ref_I] -> Inverter Pole Control (Current/Voltage/Gamma)/3(Id_ref (pu))
  On Delay (IC=1)/1 -> Inverter Pole Control (Current/Voltage/Gamma)/5(Block), 12-pulse Firing Control/3(Block)
  Enable Ref.  Voltage Step/1 -> Inverter Pole Control (Current/Voltage/Gamma)/4(Vd_ref (pu)), [Vd_ref_I]
  Vd_ref/1 -> Enable Ref.  Voltage Step/2
  Vd_ref Step/1 -> Enable Ref.  Voltage Step/1
  Monostable (IC=1)/1 -> Inverter Pole Control (Current/Voltage/Gamma)/6(Forced_alpha)
  [PulsesD_I] -> Unit Delay1/1
  Thyristor currents Y bridge/1 -> Gamma Measurement/2(I_th(1-6)_Y)
  "Thyristor currents D bridge "/1 -> Gamma Measurement/3(I_th(1-6)_D)
  Unit Delay/1 -> Gamma Measurement/5(PulsesY)
  Unit Delay1/1 -> Gamma Measurement/6(PulsesD)
  [PulsesY_I] -> Unit Delay/1
  12-pulse Firing Control/3(Freq) -> Gamma Measurement/4(Freq)
  12-pulse Firing Control/1(PulsesY) -> [PulsesY_I]
  12-pulse Firing Control/2(PulsesD) -> [PulsesD_I]

== system North_Country_Grid/Chateauguay HVDC Back-to-Back Converter/Master Control ==
  note: Master Control
  note: Balanced reference currents
  Constant : Constant  Value=0
  Enable Ref. Current Step : ManualSwitch  CurrentSetting=0
  Id_ref Step : spsStairGeneratorLib/Stair Generator  t="[ 0  0.7  0.8  ]"  e="[ 0   -0.2   0  ]"  Ts=Ts
  Informations : Subsystem
      mask Display: disp('?')
  Start/Stop : Subsystem  mask(Start/Stop  & Ramping){Min_ref=0.1, X_start=[0.3333, 0.02], X_up=[5.0, 0.4, 1.0], X_down=[-5.0,  1.4], T_stop=1.6, Ts=Ts}
      mask prompts: Min_ref "Minimum Steady-State Current Reference (pu):"; X_start "{Start Ramp}: [Rate (pu/s), Time (s)]"; X_up "{Up Ramp}: [Rate (pu/s), Time (s), Final Value (pu)]"; X_down "{Down Ramp}: [Rate (-pu/s), Time (s)]"; T_stop "Stop Time (s):"; Ts "Sample Time (s):"
      mask help:
      | At start-up, both converters are deblocked and ramped up to the minimum current (Minimum Steady-State Current Reference) with an adjustable rate (Start Ramp Rate) and application time (Start Ramp Time).
      |
      | After the system stabilisation the current is ramped up to its final value (Up Ramp Final Value) with an adjustable rate (Up Ramp Rate) and execution time (Up Ramp Time).
      |
      | Before stopping the converters (at Stop Time) the current is ramped down to the minimum current  with an adjustable rate (Down Ramp Rate) and execution time  (Down Ramp Time).
      |
      | At Stop Time the reference is ramped down to zero with the same rate used for the Start Ramp.
      mask init:
      | T_up = X_up(2); F_up = X_up(3); up_slope = X_up(1);
      | T_up_final =  T_up + (F_up - Min_ref)/up_slope;
      | 
      | T_down = X_down(2); F_down = Min_ref; down_slope = X_down(1);
      | T_down_final =   T_down + (F_down-F_up)/down_slope;
      | 
      | SS_ramp = X_start(1); T_start = X_start(2);
      | 
      | T_ramp  = [0, T_up, T_up_final,  T_down,  T_down_final, 9999]';
      | U_ramp = [0, 0, F_up-Min_ref,  F_up-Min_ref,  F_down- Min_ref,  F_down - Min_ref]';
      mask Display: disp('Start/Stop\n & Ramping')
  Sum : Sum  SaturateOnIntegerOverflow=on
  tag scope: Id_ref_I=global, Id_ref_R=global, Stop_I=global, Stop_R=global
  wires:
  Id_ref Step/1 -> Enable Ref. Current Step/1
  Constant/1 -> Enable Ref. Current Step/2
  Enable Ref. Current Step/1 -> Sum/2
  Sum/1 -> [Id_ref_R], [Id_ref_I]
  Start/Stop/2("Stop ") -> [Stop_I], [Stop_R]
  Start/Stop/1(Id_ref_ramp) -> Sum/1

== system North_Country_Grid/Chateauguay HVDC Back-to-Back Converter/Rectifier ==
  1200 MVA : spsThreePhaseTransformerThreeWindingsLib/Three-Phase Transformer (Three Windings)  Winding1Connection=Yg  Winding2Connection=Y  Winding3Connection=Delta (D1)  CoreType=Three single-phase transformers  SetSaturation=off  Hysteresis=off  DataFile='hysteresis'  SetInitialFlux=off  Measurements=None  UNITS=pu  NominalPower=[ 1200e6 , 60 ]  Winding1="[VLL_nom_R*0.9 0.0025  0 ]"  Winding2=[ 200e3 0.0025 0.24]  Winding3=[ 200e3 0.0025 0.24 ]  Rm=500  Lm=500  L0=0.5  Saturation="[0 0; 0.0024 1.2; 1.0  1.45]"  InitialFluxes=[-1.26114097729929 0.657669801639854 0.603471175659435]  BreakLoop=off  DiscreteSolver=Trapezoidal iterative  DataType=off  TransfoNumber=0
      settings: AttributesFormatString=\n
  A->pu : Gain  Gain=1/Idc_nom  SaturateOnIntegerOverflow=on  OutDataTypeStr=Inherit: Same as input  ParamDataTypeStr=Inherit: Same as input
  Rectifier : Subsystem
      mask Display: plot(0,0,100,100,[30 70 50 30 ], [40 40 60 40], [50 50], [25 40], [50 50], [ 60 75], [30 70], [60 60], [50 40 30], [60 70 70]);
  Zrec : spsImpedanceMeasurementLib/Impedance Measurement  LConnTagsString=+|-  Factor=1/2
  idR : spsCurrentMeasurementLib/Current Measurement  Tag=PoWeRsYsTeMmEaSuReMeNt  PhasorSimulation=off  OutputType=Magnitude  PSBequivalent=0
      settings: AttributesFormatString=\n
  A : PMIOPort  Side=Left
  B : PMIOPort  Port=2  Side=Left
  C : PMIOPort  Port=3  Side=Left
  "+ " : PMIOPort  Port=4  Side=Right
  - : PMIOPort  Port=5  Side=Right
  tag scope: Id_R=global
  wires:
  idR/1 -> A->pu/1
  A->pu/1 -> [Id_R]
  [PulsesY_R] -> Rectifier/1(Py)
  [PulsesD_R] -> Rectifier/2(Pd)
  connections:
  idR/RConn1 -- "+ "/RConn1
  Rectifier/RConn2 -- -/RConn1
  Rectifier/RConn1 -- idR/LConn1
  Rectifier/LConn6 -- 1200 MVA/RConn6
  1200 MVA/RConn5 -- Rectifier/LConn5
  Rectifier/LConn4 -- 1200 MVA/RConn4
  1200 MVA/RConn3 -- Rectifier/LConn3
  Rectifier/LConn2 -- 1200 MVA/RConn2
  1200 MVA/RConn1 -- Rectifier/LConn1
  A/RConn1 -- Zrec/LConn1 -- 1200 MVA/LConn1
  B/RConn1 -- Zrec/LConn2 -- 1200 MVA/LConn2
  C/RConn1 -- 1200 MVA/LConn3

== system North_Country_Grid/Chateauguay HVDC Back-to-Back Converter/Rectifier Control and Protection ==
  note: Block/Deblock sequence
  12-pulse Firing Control : Subsystem  mask(HVDC Discrete 12-pulse Firing Control){Pw=101.5, PLL_PF=[0,  Fnom_R], PLL_G=[60, 1400], dt=Ts}
      mask prompts: Pw "{Pulse Generator}: Pulse Width (deg)"; PLL_PF "{PLL}: Initial [Phase (deg) Frequency (Hz)]"; PLL_G "{PLL}: Regulator gains [Kp (rad)  Ki (rad/s)]"; dt "Sample Time (s):"
      mask help:
      | This block contains a PLL and a 12-pulse generator to provide the firing pulses to the HVDC converter.
      | The firing control is of the equidistant type. It is based on a Phase Locked Loop (PLL) synchronized on positive-sequence of the fundamental voltage.
      mask init:
      | PLL_ph = PLL_PF(1); PLL_f0 = PLL_PF(2);
      | PLL_Kp = PLL_G(1); PLL_Ki = PLL_G(2);
      mask Help:
      | INPUTS:
      | alpha :  Desired firing angle of thyristors (deg).
      | Vabc  : 3 phase-to-ground voltages (pu)  on the primary winding of the YgYD converter transformer
      | Block  : Logical signal  (0-1). The pulses are not generated when the value is 1.
      | 
      | 
      | 
      | OUTPUTS:
      |  PulsesY :  6 pulses to be sent to the half converter connected to the Wye winding.
      |  PulsesD :  6 pulses to be sent to the half converter connected to the Delta winding.
  Data Type Conversion : DataTypeConversion  OutDataTypeStr=boolean
  Ground : Ground
  Logical Operator2 : Logic  Operator=OR  AllPortsSameDT=off
  Logical Operator3 : Logic  Operator=NOT
  Monostable : spsMonostableLib/Monostable  EdgeDetect=Rising  PulseDuration=0.15  ic=1  Ts=Ts
  Multimeter : spsMultimeterLib/Multimeter  Tag=PoWeRsYsTeMmEaSuReMeNt  L=44  sel=21  yselected={}  Gain=1  OutputType=Magnitude  PlotAtSimulationStop=off  PhasorSimulation=off
      settings: AttributesFormatString=\n
  On Delay : spsOnDelayLib/On Delay  DelayType=On delay  delay=0.1  ic=1  Ts=Ts
  Rectifier Pole Control (Current) : Subsystem  DialogController=POWERSYS.PowerSysDialog  mask(Discrete HVDC Controller){Mode=Rectifier (Current), XPILim=[166, 5], XLin=[160, 120], XKPI_I=[45, 4500, 90], Id_marg=0.1, XKPI_V=[35, 2250,  90], Vd_marg=0.05, XKPI_G=[1, 20,  90 ], G_marg=1, T_I=0.3e-3, XT_V=[15,  0.707], Xvdcol=[0.6, 0.18, 0.30, 0.1, 0.080], alpha_const=off, Xalpha_fix=[166, inf, -inf], Ts=Ts}
      mask prompts: Mode "Control Mode :"; XPILim "{Alpha Limits}  [alpha max (deg), alpha min (deg) ]"; XLin "Kp Lin. Angle Limits (alpha or beta) : [Max  (deg), Min  (deg) ]"; XKPI_I "{Current Regulator}   [Kp (deg/pu) , Ki (deg/pu/s), AlphaInit (deg) ]"; Id_marg "Current Margin (pu) :"; XKPI_V "{Voltage Regulator}   [Kp (deg/pu) , Ki (deg/pu/s),  AlphaInit (deg) ]"; Vd_marg "Voltage Margin (pu):"; XKPI_G "{Gamma Regulator} [Kp, Ki (s), AlphaInit (deg)]"; G_marg "Gamma Margin (deg):"; T_I "{Id Meas. Filter H(s)=1/(1+Ts)} T(s):"; XT_V "{Vd Meas. Low-Pass 2nd Order Filter}  [fo,  Zeta ]"; Xvdcol "{VDCOL}  [ VdThresh.(pu),VdMin(pu),IdMin(pu),IdMinAbs(pu),Tup(s) ]"; alpha_const "Constant alpha mode"; Xalpha_fix "{Ct.  or Forced alpha)}  [Alpha (deg), + Rate limit, - Rate limit (deg/s)]"; Ts "Sample Time (s):"
      mask help:
      | This block contains the regulators and functions to control the firing angle alpha of a HVDC rectifier or inverter.
      |  See the 'HVDC Transmission System' case study of the User's Manual for description of the block functionality.
      mask init: same as North_Country_Grid/Chateauguay HVDC Back-to-Back Converter/Inverter Control and Protection/Inverter Pole Control (Current/Voltage/Gamma)
      mask Help: This block is part of a subset of blocks in the Extras library that does not have documentation associated with it, other than the block mask description.
      mask TypeOptions Mode: Rectifier (Current) | Inverter (Current + Voltage + Gamma) | Inverter (Current + Voltage) | Inverter (Current + Gamma)
      mask Callback Mode:
      | mode=get_param(gcb,'Mode');
      | 
      | cb=get_param(gcb,'MaskVisibilities');
      | 
      | if strcmp(mode,'Rectifier (Current)')
      | 	cb{10}='on';
      |     cb{11} = 'off';
      | 
      | 	 cb{3}='off';
      | 	 cb{5}='off';cb{6}='off';cb{7}='off';cb{8}='off';cb{9}='off';
      |     set_param(gcb,'MaskVisibilities',cb);
      | elseif (strcmp(mode,'Inverter (Current + Voltage + Gamma)'))
      | 	 cb{3}='off';
      | 	 cb{5}='on';cb{6}='on';cb{7}='on';cb{8}='on';cb{9}='on';cb{11} = 'on';
      | 	 set_param(gcb,'MaskVisibilities',cb);
      | elseif (strcmp(mode,'Inverter (Current + Voltage)'))
      | 	 cb{3}='off';
      | 	 cb{5}='on';cb{6}='on';cb{7}='on';cb{8}='off';cb{9}='off'; cb{11} = 'on';
      |      set_param(gcb,'MaskVisibilities',cb);
      | else
      | 	 cb{3}='off';
      | 	 cb{5}='on';cb{6}='off';cb{7}='off';cb{8}='on';cb{9}='on'; cb{11} = 'on';
      | 	 set_param(gcb,'MaskVisibilities',cb);
      | end
      mask Display: disp('')
  Rectifier Protections : Subsystem  TreatAsAtomicUnit=on  mask(Protection LACVD a Radisson (cyc = 1 ms)){}
  Terminator : Terminator
  V->pu : Gain  Gain=1/Vdc_nom  SaturateOnIntegerOverflow=on  OutDataTypeStr=Inherit: Same as input  ParamDataTypeStr=Inherit: Same as input
  tag scope: Forced_alpha_R=global, Id_ref_lim_R=global, Low_ac_volt_R=global, Mode_R=global, PulsesD_R=global, PulsesY_R=global, VdL_R=global, alpha_ord_R=global
  wires:
  [Low_ac_volt_I] -> Rectifier Protections/4(Low_ac_volt_oth)
  Rectifier Protections/2(Low_ac_voltage) -> [Low_ac_volt_R]
  Monostable/1 -> Logical Operator2/1
  On Delay/1 -> 12-pulse Firing Control/3(Block), Rectifier Pole Control (Current)/5(Block), Logical Operator3/1
  Rectifier Protections/1(Forced_alpha) -> Logical Operator2/2
  Data Type Conversion/1 -> On Delay/1, Monostable/1
  [Vabc_R] -> Rectifier Protections/1(Uabc (pu))
  [VdL_R] -> Rectifier Protections/2(VdL (pu))
  Logical Operator3/1 -> Rectifier Protections/3(Deblocked)
  [Stop_R] -> Data Type Conversion/1
  Ground/1 -> Rectifier Pole Control (Current)/9(D_alpha (deg)), Rectifier Pole Control (Current)/8(gamma_ref (deg)), Rectifier Pole Control (Current)/7(gamma_meas (deg)), Rectifier Pole Control (Current)/4(Vd_ref (pu))
  [VdL_R] -> Rectifier Pole Control (Current)/1(VdL (pu))
  [Id_R] -> Rectifier Pole Control (Current)/2(Id (pu))
  Rectifier Pole Control (Current)/1(alpha_ord (deg)) -> 12-pulse Firing Control/1(alpha_ord (deg)), [alpha_ord_R]
  Rectifier Pole Control (Current)/2(Id_ref_lim) -> [Id_ref_lim_R]
  Rectifier Pole Control (Current)/3(mode) -> [Mode_R]
  Logical Operator2/1 -> Rectifier Pole Control (Current)/6(Forced_alpha), [Forced_alpha_R]
  Multimeter/1 -> V->pu/1  "Vd Line"
  V->pu/1 -> [VdL_R]
  [Id_ref_R] -> Rectifier Pole Control (Current)/3(Id_ref (pu))
  12-pulse Firing Control/1(PulsesY) -> [PulsesY_R]
  [Vabc_R] -> 12-pulse Firing Control/2(Vabc (pu))
  12-pulse Firing Control/2(PulsesD) -> [PulsesD_R]
  12-pulse Firing Control/3(Freq) -> Terminator/1
